simulink model "LOD"  (R2018a)
settings: Solver=VariableStepAuto  StartTime=0.0  StopTime=30  RelTol=1e-3
settings Model: Creator=86153  LastModifiedBy=86153

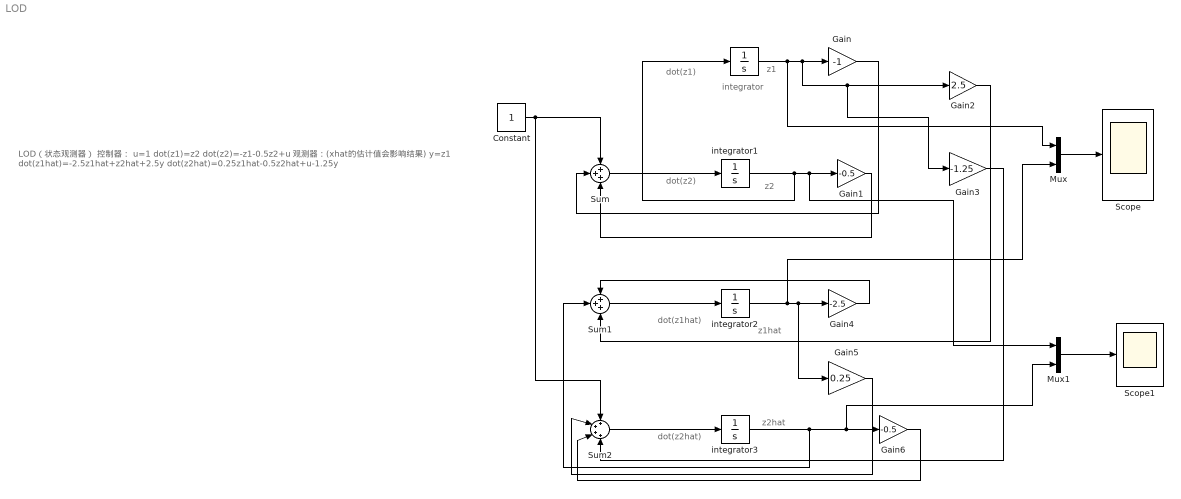
== system LOD ==
  note: LOD（状态观测器）
      | 控制器：
      | u=1
      | dot(z1)=z2
      | dot(z2)=-z1-0.5z2+u
      |
      | 观测器：(xhat的估计值会影响结果)
      | y=z1
      | dot(z1hat)=-2.5z1hat+z2hat+2.5y
      | dot(z2hat)=0.25z1hat-0.5z2hat+u-1.25y
  note: integrator
  note: z1hat
  note: z2
  note: dot(z1)
  note: z1
  note: dot(z2)
  note: dot(z1hat)
  note: z2hat
  note: dot(z2hat)
  " " : Integrator
  Constant : Constant
  Gain : Gain  Gain=-1
  Gain1 : Gain  Gain=-0.5
  Gain2 : Gain  Gain=2.5
  Gain3 : Gain  Gain=-1.25
  Gain4 : Gain  Gain=-2.5
  Gain5 : Gain  Gain=0.25
  Gain6 : Gain  Gain=-0.5
  Mux : Mux  Inputs=2
  Mux1 : Mux  Inputs=2
  Scope : Scope
  Scope1 : Scope
  Sum : Sum  Inputs=+++
  Sum1 : Sum  Inputs=+++
  Sum2 : Sum  Inputs=++++
  integrator1 : Integrator
  integrator2 : Integrator
  integrator3 : Integrator  InitialCondition=1
  wires:
  integrator1/1 -> Mux1/1, Gain1/1, " "/1
  " "/1 -> Mux/1, Gain3/1, Gain2/1, Gain/1
  Gain1/1 -> Sum/3
  Gain/1 -> Sum/2
  Sum/1 -> integrator1/1
  Constant/1 -> Sum2/1, Sum/1
  Gain2/1 -> Sum1/3
  integrator3/1 -> Sum1/2, Mux1/2, Gain6/1
  Gain4/1 -> Sum1/1
  integrator2/1 -> Mux/2, Gain5/1, Gain4/1
  Gain3/1 -> Sum2/4
  Gain6/1 -> Sum2/3
  Gain5/1 -> Sum2/2
  Sum1/1 -> integrator2/1
  Sum2/1 -> integrator3/1
  Mux1/1 -> Scope1/1
  Mux/1 -> Scope/1
